simulink model "Aplicacion"  (Simulink 9.1)
settings: Solver=ode45  StartTime=0.0  StopTime=30  RelTol=1e-3  AbsTol=1e-6
values from neighbouring files (symbols this model uses):
  b0 = 3    [sys.m]
  b1 = 3    [sys.m]
  b2 = 4    [sys.m]
  b3 = 2    [sys.m]
  k = 3    [sys.m]
undefined symbols (not defined in the file or in its folder): sfunxy2
libraries: neural x1
settings Model: SuppressorTable=22 serialization::archive 11 0 6 0 0 0 1 0  Creator=munlock -all d:\work\myr12\toolbox\fuzzy\fuzzy\mfedit.m  LastModifiedBy=daniel  ExtModeTrigMode=oneshot  ExtModeArmWhenConnect=off  TunableVars=prueba  TunableVarsStorageClass=Auto
settings SolverCC: AutoScaleAbsTol=off
settings DataIOCC: SignalLoggingSaveFormat=ModelDataLogs  SaveOutput=off  SignalLoggingName=sigsOut
settings OptimizationCC: BooleanDataType=off  InitFltsAndDblsToZero=on
settings DebuggingCC: SaveWithParameterizedLinksMsg=none  SignalResolutionControl=TryResolveAllWithWarning  MultiTaskDSMMsg=warning  MultiTaskCondExecSysMsg=none
settings HardwareCC: TargetUnknown=on
settings RTWCC: TemplateMakefile=grt_vc.tmf
settings GRTTargetCC: TargetFcnLib=ansi_tfl_tmw.mat

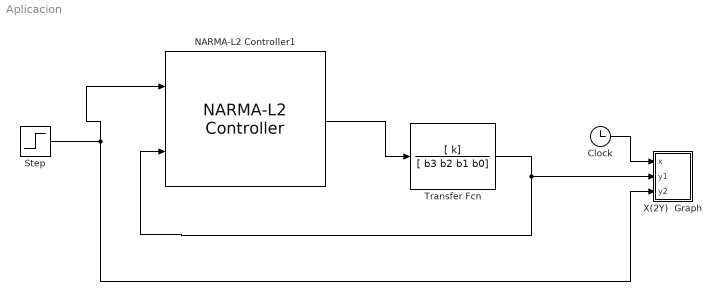
== system Aplicacion ==
  Clock : Clock
  NARMA-L2 Controller1 : neural/Control Systems/NARMA-L2 Controller  Normalize=1  IW1_1=[1.7230491874233626604 -0.41072126168373507271 -0.20223517008692398766 -0.0091724441425070669942 -0.007181452027622609556;0.3819567361242267034 0.50864306402961734221 -0.46285339003047382134 -0.00028515592580728943645 0.00015591257192208984048;0.014782738311384822569 -1.8466835271436525812 0.89587025235226536157 0.017162423438475214038 0.016461184711729203584]  IW3_2=[1.873583666471571707 -0.70010603726794384816 0.24513646818650960957 -0.0041377898220113038669 -0.0041421819500487531973;-0.57517030993258089211 -1.8256685096096152421 0.66340109678701164597 -0.036741141400521884486 -0.03682652912770990189;1.9859039946370060647 -0.43209683136185345065 0.1901793857895213713 -0.0065705052450540117268 -0.0065740492106202558231]  IW5_3=0.41000528061972268956  LW2_1=[-0.42201721252753576774 -1.6027197766196927819 -0.57778441910835676154]  LW4_3=[-0.39360708607058475517 -0.70317054553334989997 -0.68799436239365208134]  LW5_4=-0.0080592038734365739616  LW6_5=0.39173421266264113472  LW6_2=-1.429751599673434459  B1=[-1.4341525970831101588;0.28392380404957484608;2.1118258273934804592]  B2=0.62711444266918836554  B3=[-2.0247004964021719786;-0.045218654470003095958;2.0056585797765626999]  B4=-0.69317051564884168968  Limit_output=0  min_output=-Inf  max_output=Inf  Use_Previous_Weights=1  Ts=0.03  S1=3  Ni=3  Nj=3  sim_file=ModeloPlanta  trainfun=trainlm  Use_validation=1  Use_Testing=1  max_i=10  min_i=0  max_i_int=10  min_i_int=1  sam_training=800  epochs=1200  minp=5.0595705166514237661  maxp=9.5974395851608100827  mint=0  maxt=9.5974395851608100827
      settings: SourceProductName=Neural Network Toolbox  SourceProductBaseCode=NN
  Step : Step  Time=0  SampleTime=0
  Transfer Fcn : TransferFcn  Numerator=[ k]  Denominator=[ b3 b2 b1 b0]
  X(2Y)  Graph : Subsystem  LoadFcn=sfunxy2([],[],[],'LoadBlock')  StartFcn=sfunxy2([],[],[],'Start')  StopFcn=sfunxy2([],[],[],'Stop')  mask(X(2Y) scope.){xmin=0, xmax=10, ymin=0, ymax=2, st=-1}
      mask prompts: xmin "x-min:"; xmax "x-max:"; ymin "y-min:"; ymax "y-max:"; st "Sample time:"
      mask help: X(2Y) scope using MATLAB graph window. First input is used as time base. Enter plotting ranges.
      settings: CopyFcn=sfunxy2([],[],[],'CopyBlock')  DeleteFcn=sfunxy2([],[],[],'DeleteBlock')  NameChangeFcn=sfunxy2([],[],[],'NameChange')
      mask Help: This block can be used to explore limit cycles. Look at the m-file sfunxy.m to see how it works.
      mask Display: plot([.05 .95 .95 .05 .05],[.45 .45 .95 .95 .45], 0.5+cos(0:0.1:2*pi)*0.3,0.7+sin(0:0.1:2*pi)*0.2)
  wires:
  Clock/1 -> X(2Y)  Graph/1(x)
  Step/1 -> NARMA-L2 Controller1/1, X(2Y)  Graph/3(y2)
  Transfer Fcn/1 -> NARMA-L2 Controller1/2, X(2Y)  Graph/2(y1)
  NARMA-L2 Controller1/1 -> Transfer Fcn/1

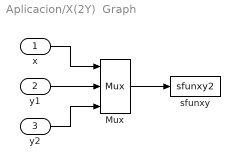
== system Aplicacion/X(2Y)  Graph ==
  x : Inport
  y1 : Inport  Port=2
  y2 : Inport  Port=3
  Mux : Mux  Inputs=3
  sfunxy : S-Function  FunctionName=sfunxy2  Parameters=[xmin xmax ymin ymax], st  SFunctionDeploymentMode=off  EnableBusSupport=off
  wires:
  y2/1 -> Mux/3
  y1/1 -> Mux/2
  x/1 -> Mux/1
  Mux/1 -> sfunxy/1
